simulink model "Traditional_Flyback_RC"  (R2015a)
settings: Solver=ode45  SolverMode=SingleTasking  StartTime=0.0  StopTime=0.002  FixedStep=1e-10  RelTol=1e-3
libraries: powerlib x9
settings Model: SimulationMode=accelerator  CovMetricSettings=dwe  CovHtmlReporting=off  covSaveCumulativeToWorkspaceVar=off  CovSaveSingleToWorkspaceVar=off  CovExternalEMLEnable=on  Creator=vibra  LastModifiedBy=vibra
settings DataIOCC: LimitDataPoints=off  SaveFormat=Dataset  ReturnWorkspaceOutputs=on
settings DebuggingCC: SFUnexpectedBacktrackingDiag=error  SFNoUnconditionalDefaultTransitionDiag=error
settings HardwareCC: ProdBitPerPointer=64  ProdLargestAtomicFloat=Float  ProdIntDivRoundTo=Zero  ProdEndianess=LittleEndian  ProdHWDeviceType=Specified
settings ModelReferenceCC: PropagateSignalLabelsOutOfModel=on
settings SFSimCC: SimUseLocalCustomCode=on
settings RTWCC: RTWUseLocalCustomCode=on
settings GRTTargetCC: TargetLangStandard=C99 (ISO)  GeneratePreprocessorConditionals=Use local settings
settings ConfigurationSet: Description=Simscape Multibody

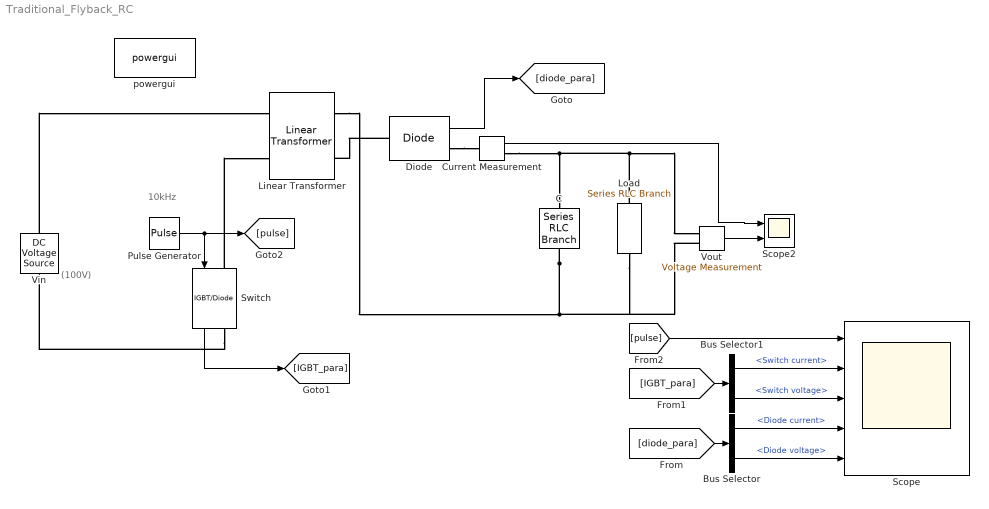
== system Traditional_Flyback_RC ==
  note: (100V)
  note: 10kHz
  Bus Selector : BusSelector  OutputSignals=Diode current,Diode voltage
  Bus Selector1 : BusSelector  OutputSignals=Switch current,Switch voltage
  C : powerlib/Elements/Series RLC Branch  LConnTagsString=__new0  RConnTagsString=__new0  BranchType=C  Resistance=1e-4  Inductance=200e-6  SetiL0=off  InitialCurrent=0  Capacitance=200e-5  Setx0=off  InitialVoltage=0  Measurements=None
  Current Measurement : powerlib/Measurements/Current Measurement  PhasorSimulation=off  OutputType=Complex  PSBequivalent=0
  Diode : powerlib/Power Electronics/Diode  Ron=0.001  Lon=0  Vf=0.8  IC=0  UseSnubber=0  Rs=500  Cs=250e-9  Measurements=on
  Linear Transformer : powerlib/Elements/Linear Transformer  UNITS=SI  NominalPower=[ 25 100e3 ]  winding1=[150 0 10e-9]  winding2=[30 0 0]  ThreeWindings=off  winding3=[3.15e+05 3.969e+07 6316.9]  RmLm=[10000 300e-6]  Measurements=Magnetization current  DataType=on
  Load : powerlib/Elements/Series RLC Branch  LConnTagsString=__new0  RConnTagsString=__new0  BranchType=R  Resistance=10  Inductance=200e-6  SetiL0=off  InitialCurrent=0  Capacitance=400e-6  Setx0=off  InitialVoltage=0  Measurements=Branch current
  Pulse Generator : DiscretePulseGenerator  PulseType=Time based  Period=1/100e2  PulseWidth=30
  Scope : Scope  NumInputPorts=5
      settings: TimeRange=auto  ShowLegends=on  MaxDataPoints=5000  SaveToWorkspace=off  SaveName=ScopeData  YMin=-0.125~-44.0642~-6.65795~-75.34483~-75.34483  YMax=1.125~396.15907~230.4692~284.86261~284.86261  SampleTime=-1
  Scope2 : Scope  NumInputPorts=2
      settings: TimeRange=auto  MaxDataPoints=5000  SaveToWorkspace=off  SaveName=ScopeData2  YMin=36.77863~-7.21778  YMax=163.15601~64.8787  SampleTime=-1
  Switch : powerlib/Power Electronics/IGBT//Diode  Ron=1e-6  Rs=1e-6  Cs=1e-9  Measurements=on
  Vin : powerlib/Electrical Sources/DC Voltage Source  Amplitude=100  Measurements=None
  Vout : powerlib/Measurements/Voltage Measurement  PhasorSimulation=off  OutputType=Complex  PSBequivalent=0
  powergui : powerlib/powergui  Priority=1  SimulationMode=Discrete  SampleTime=5e-10  frequency=60  Iterations=50  frequencyindice=0  Pbase=100e6  ErrMax=1e-4  UnitsV=kV  UnitsW=MW  buscounter=0  FunctionMessages=off  echomessages=off  EnableUseOfTLC=off  CurrentSourceSwitches=off  DisableSnubberDevices=off  DisableRonSwitches=off  DisableVfSwitches=off  DisplayEquations=off  AutomaticDiscreteSolvers=off  SolverType=Tustin/Backward Euler (TBE)  Interpol=off  ExternalGateDelay=off  methode=off  Ts=100  x0status=blocks  SPID=on  SwTol=0  HookPort=off  NonlinearTolerance=0  nMaxIteration=15  ContinueOnMaxIteration=off  RestoreLinks=warning  ResistiveCurrentMeasurement=off  Frange=[0:2:500]  Ylog=off  Xlog=on  ShowGrid=off  save=off  variable=ZData  structure=0  ZoomFFT=off  StartTime=0.0  cycles=1  DisplayStyle=1  fundamental=60  FreqAxis=off  MaxFrequency=1000  frequencyindicesteady=1  RmsSteady=1  display=off
  wires:
  [pulse] -> Scope/1
  Pulse Generator/1 -> Switch/1, [pulse]
  Switch/1 -> [IGBT_para]
  Diode/1 -> [diode_para]
  Vout/1 -> Scope2/2
  Current Measurement/1 -> Scope2/1
  [diode_para] -> Bus Selector/1
  Bus Selector/1 -> Scope/4  "<Diode current>"
  Bus Selector/2 -> Scope/5  "<Diode voltage>"
  [IGBT_para] -> Bus Selector1/1
  Bus Selector1/1 -> Scope/2  "<Switch current>"
  Bus Selector1/2 -> Scope/3  "<Switch voltage>"
  connections:
  C/RConn1 -- Linear Transformer/RConn1 -- Load/RConn1 -- Vout/LConn2
  Switch/LConn1 -- Linear Transformer/LConn2
  Load/LConn1 -- Current Measurement/RConn1 -- C/LConn1 -- Vout/LConn1
  Vin/RConn1 -- Linear Transformer/LConn1
  Switch/RConn1 -- Vin/LConn1
  Diode/LConn1 -- Linear Transformer/RConn2
  Diode/RConn1 -- Current Measurement/LConn1
